simulink model "WL_test"  (R2025a)
settings: Solver=ode4  StartTime=0.0  StopTime=T_sim  FixedStep=Dt_sim  RelTol=1e-3
InitFcn:
  | % --- AVVIO AUTOMATICO PYTHON SERVER CON POP-UP (METODO FILE ROBUSTO) ---
  | fprintf('[Simulink] Preparazione simulazione...\n');
  | 
  | % 1. Pop-up per la Raffica
  | scelta_gust = questdlg('Vuoi includere la gust?', ...
  |     'Configurazione Raffica', 'Si', 'No', 'No');
  | if isempty(scelta_gust), scelta_gust = 'No'; end
  | 
  | % 2. Pop-up per il Video
  | scelta_video = questdlg('Vuoi generare il video MP4 a fine simulazione?', ...
  |     'Configurazione Video', 'Si', 'No', 'No');
  | if isempty(scelta_video), scelta_video = 'No'; end
  | 
  | % --- PERCORSO ASSOLUTO ---
  | % Definiamo subito la cartella così MATLAB e WSL salvano e leggono dallo stesso posto
  | percorso = '/home/lpmatteo/software/WingLoop/WingLoop_Library/wingloop_testrun/';
  | file_inputs = fullfile(percorso, 'python_inputs.txt');
  | 
  | % --- CREAZIONE FILE DI INPUT ---
  | fid = fopen(file_inputs, 'w');
  | fprintf(fid, '1\n'); % Scelta controller: 1 (LQI)
  | 
  | if strcmp(scelta_gust, 'Si')
  |     fprintf(fid, 's\n');
  | else
  |     fprintf(fid, 'n\n');
  | end
  | 
  | if strcmp(scelta_video, 'Si')
  |     % Se vogliamo il video, precompiliamo anche formato (mp4), qualità (high)
  |     % e la "Y" finale per far partire il render ASWING in automatico.
  |     fprintf(fid, 's\ngif\nmedium\nY\n');
  | else
  |     fprintf(fid, 'n\n');
  | end
  | fclose(fid);
  | 
  | % --- AVVIO DEL SERVER WSL ---
  | % Diciamo a Python di prendere le risposte direttamente dal file appena creato
  | cmd_wsl = sprintf('start "WingLoop Python Server" wsl -e bash -ic "cd %s && conda activate WINGLOOP && python3 controller_wingloop.py < python_inputs.txt; exec bash"', percorso);
  | 
  | system(cmd_wsl);
values from neighbouring files (symbols this model uses):
  Dt_asw = 0.1    [WL_main.m]
  u_trim = [0, F2ref, F3ref, 0, E2ref, E2ref]    [WL_main.m]
undefined symbols (not defined in the file or in its folder): FullModel
settings Model: SimulationMode=accelerator  Creator=lpmat  LastModifiedBy=lpmat

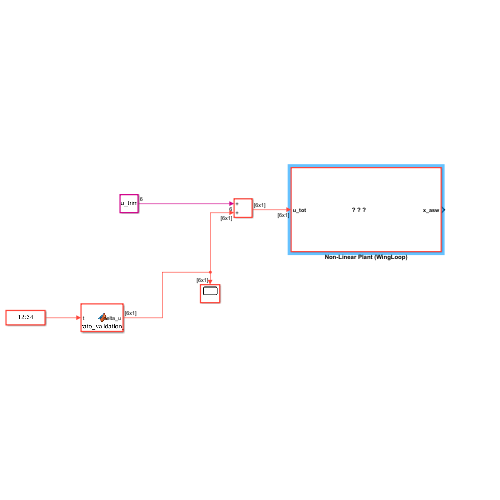
[thumbnail: Simulink's stored preview of the top-level diagram]
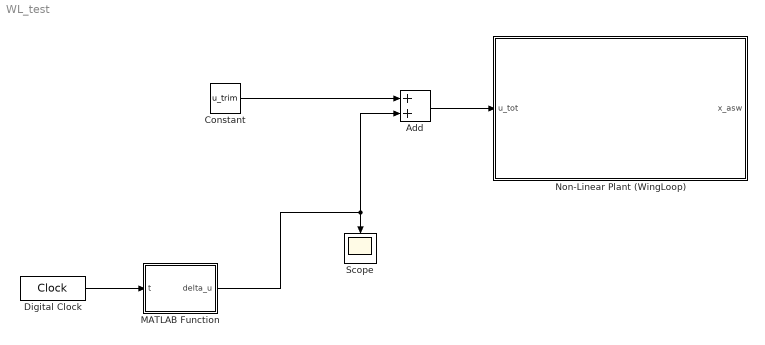
== system WL_test ==
  Add : Sum
  Constant : Constant  Value=u_trim
  Digital Clock : DigitalClock  SampleTime=Dt_asw
  MATLAB Function : MATLAB Function  TreatAsAtomicUnit=on
  Non-Linear Plant (WingLoop) : Subsystem
      mask Display: image('Screenshot 2026-03-18 123158.png');
  Scope : Scope
      settings: ActiveDisplayYMinimum=-1  ActiveDisplayYMaximum=1
  wires:
  Constant/1 -> Add/1
  Add/1 -> Non-Linear Plant (WingLoop)/1(u_tot)
  Digital Clock/1 -> MATLAB Function/1(t)
  MATLAB Function/1(delta_u) -> Add/2, Scope/1

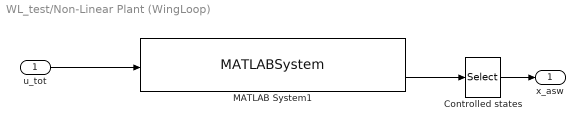
== system WL_test/Non-Linear Plant (WingLoop) ==
  u_tot : Inport
  Controlled states : Selector  InputPortWidth=1888  IndexOptions=Index vector (dialog)  Indices=[1:1882]  OutputSizes=1
  MATLAB System1 : MATLABSystem  System=AswingPlant  ServerHost=localhost  ServerPort=5005  NumModalStates=ROM.n_modal  NumPhysicalStates=FullModel.n_orig+ FullModel.n_in  SimulateUsing=Interpreted execution
      mask Type: AswingPlant
  x_asw : Outport
  wires:
  MATLAB System1/2 -> Controlled states/1
  u_tot/1 -> MATLAB System1/1
  Controlled states/1 -> x_asw/1

== matlab function WL_test/MATLAB Function ==
  data: t input; delta_u output
function delta_u = generate_validation_cmd(t)
    % Parametri della manovra
    t_start = 1.0;  % Inizio incremento a 1 secondo
    tau = 1.0;      % Costante di tempo (velocità della curva)
    
    % Inizializziamo il vettore delta_u (6 canali)
    delta_u = zeros(6, 1);
    
    if t >= t_start
        % Calcolo della dinamica esponenziale: 1 - exp(-t/tau)
        % Arriva al 99% del target in circa 5*tau secondi
        dinamica = (1.0 - exp(-(t - t_start) / tau));
        
        % Canale 2: Flap (+1 grado)
        delta_u(2) = 1.0 * dinamica;
        
        
    end
end
